simulink model "zad1"  (R2017a)
settings: Solver=VariableStepAuto  StartTime=0.0  StopTime=16  RelTol=1e-3
settings Model: Creator=DoktorHax  LastModifiedBy=DoktorHax

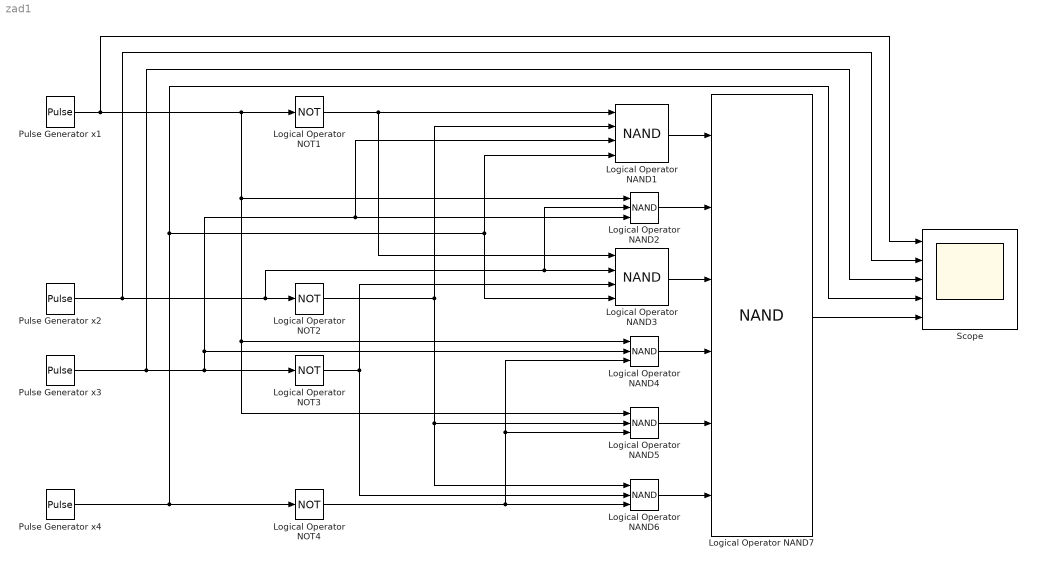
== system zad1 ==
  Logical Operator NAND1 : Logic  Operator=NAND  Inputs=4  AllPortsSameDT=off  OutDataTypeStr=boolean
  Logical Operator NAND{2,4..6} (4 alike) : Logic  Operator=NAND  Inputs=3  AllPortsSameDT=off  OutDataTypeStr=boolean
  Logical Operator NAND3 : Logic  Operator=NAND  Inputs=4  AllPortsSameDT=off  OutDataTypeStr=boolean
  Logical Operator NAND7 : Logic  Operator=NAND  Inputs=6  AllPortsSameDT=off  OutDataTypeStr=boolean
  Logical Operator NOT{1..4} (4 alike) : Logic  Operator=NOT  AllPortsSameDT=off  OutDataTypeStr=boolean
  Pulse Generator x1 : DiscretePulseGenerator  PulseType=Time based  PulseWidth=50
  Pulse Generator x2 : DiscretePulseGenerator  PulseType=Time based  Period=4  PulseWidth=50
  Pulse Generator x3 : DiscretePulseGenerator  PulseType=Time based  Period=8  PulseWidth=50
  Pulse Generator x4 : DiscretePulseGenerator  PulseType=Time based  Period=16  PulseWidth=50
  Scope : Scope  NumInputPorts=5
  wires:
  Pulse Generator x1/1 -> Logical Operator NAND5/1, Logical Operator NAND4/1, Logical Operator NAND2/1, Logical Operator NOT1/1, Scope/1
  Pulse Generator x2/1 -> Logical Operator NOT2/1, Logical Operator NAND3/2, Logical Operator NAND2/2, Scope/2
  Pulse Generator x3/1 -> Logical Operator NOT3/1, Logical Operator NAND4/2, Logical Operator NAND2/3, Logical Operator NAND1/3, Scope/3
  Pulse Generator x4/1 -> Scope/4, Logical Operator NAND3/4, Logical Operator NAND1/4, Logical Operator NOT4/1
  Logical Operator NOT1/1 -> Logical Operator NAND1/1, Logical Operator NAND3/1
  Logical Operator NOT2/1 -> Logical Operator NAND1/2, Logical Operator NAND5/2, Logical Operator NAND6/1
  Logical Operator NOT3/1 -> Logical Operator NAND6/2, Logical Operator NAND3/3
  Logical Operator NOT4/1 -> Logical Operator NAND5/3, Logical Operator NAND4/3, Logical Operator NAND6/3
  Logical Operator NAND1/1 -> Logical Operator NAND7/1
  Logical Operator NAND2/1 -> Logical Operator NAND7/2
  Logical Operator NAND3/1 -> Logical Operator NAND7/3
  Logical Operator NAND4/1 -> Logical Operator NAND7/4
  Logical Operator NAND5/1 -> Logical Operator NAND7/5
  Logical Operator NAND6/1 -> Logical Operator NAND7/6
  Logical Operator NAND7/1 -> Scope/5
